simulink model "ML_receiver"  (R2016b)
settings: Solver=VariableStepDiscrete  StartTime=0.0  StopTime=inf  RelTol=1e-3
values from neighbouring files (symbols this model uses):
  avett = exp(1i*2*pi*[0:M-1]/M)    [ML_receiver_matlab.m]
  M = 8    [ML_receiver_matlab.m]    (also in MSE_matlab2.m = 16; OFDM1.m = 64; adaptive_equalization.m = 16)
  T = 1    [ML_receiver_matlab.m]    (also in optimum_filter3.m)
  W = 100/T    (= 100)    [ML_receiver_matlab.m]
libraries: commchan3 x1, commsink2 x1, commrandsrc3 x1, dspstat3 x1, simulink x1
settings Model: Creator=Shu  LastModifiedBy=Shu
settings DataIOCC: LimitDataPoints=on  SaveOutput=off  SaveTime=off
settings OptimizationCC: BooleanDataType=off  DefaultParameterBehavior=Inlined  LocalBlockOutputs=off  LifeSpan=inf
settings DebuggingCC: AlgebraicLoopMsg=error  MultiTaskRateTransMsg=warning  AllowSymbolicDim=off  SFUnexpectedBacktrackingDiag=warning  SFNoUnconditionalDefaultTransitionDiag=warning  SFExecutionAtInitializationDiag=none
settings GRTTargetCC: TargetLangStandard=C89/C90 (ANSI)  GeneratePreprocessorConditionals=Disable all
settings ConfigComp: CovMetricSettings=dw  CovHtmlReporting=on  CovSaveCumulativeToWorkspaceVar=on  CovSaveSingleToWorkspaceVar=on  CovExternalEMLEnable=off  CovSFcnEnable=off

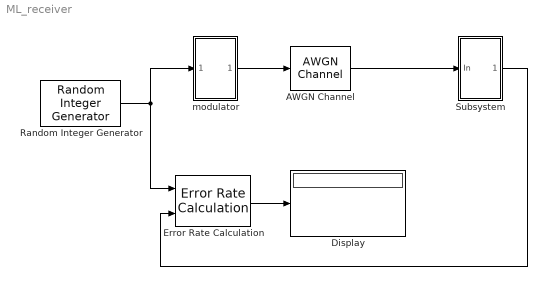
== system ML_receiver ==
  AWGN Channel : commchan3/AWGN Channel  InputProcessing=Columns as channels (frame based)  seed=67  noiseMode="Signal to noise ratio  (Es/No)"  EbNodB=10  EsNodB=SNRdB  SNRdB=SNRdB  bitsPerSym=1  Ps=1  Tsym=1  variance=1
  Display : Display
  Error Rate Calculation : commsink2/Error Rate Calculation  N=1  st_delay=1  cp_mode=Select samples from mask  subframe=[]  PMode=Port  WsName=ErrorVec  RsMode2=off  stop=off  numErr=100  maxBits=1e6
  Random Integer Generator : commrandsrc3/Random Integer Generator  SetSize=M  SeedSource=Auto  Seed=0  SampleTime=T  SamplesPerFrame=1  OutputDataType=double  SimulateUsing=Interpreted execution
  Subsystem : Subsystem
  "modulator " : Subsystem
  wires:
  Random Integer Generator/1 -> Error Rate Calculation/1, "modulator "/1(In1)
  Subsystem/1(Out1) -> Error Rate Calculation/2
  "modulator "/1(Out1) -> AWGN Channel/1
  AWGN Channel/1 -> Subsystem/1(In)
  Error Rate Calculation/1 -> Display/1

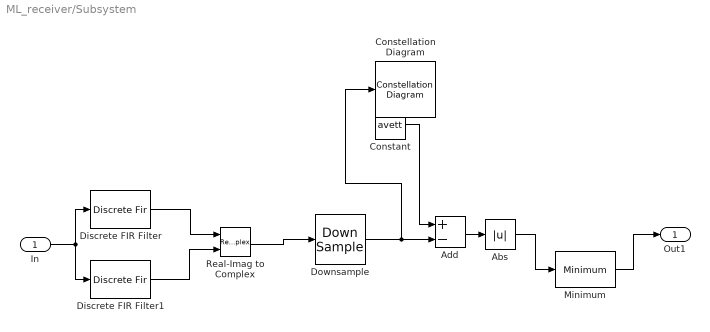
== system ML_receiver/Subsystem ==
  In : Inport
  Abs : Abs
  Add : Sum  Inputs=+-
  Constant : Constant  Value=avett  SampleTime=T
  Constellation Diagram : ConstellationDiagram
  Discrete FIR Filter : DiscreteFir  Coefficients=-sqrt(2/T)*cos(2*pi*((-W+1):0)/W)/W  InputProcessing=Columns as channels (frame based)
  Discrete FIR Filter1 : DiscreteFir  Coefficients=-sqrt(2/T)*sin(2*pi*((-W+1):0)/W)/W  InputProcessing=Columns as channels (frame based)
  Downsample : DownSample  N=W  phase=W-1  RateOptions=Allow multirate processing
  Minimum : dspstat3/Minimum  operation=minimum  fcn=Index  indexBase=Zero  operateOver=Each column  Dimension=1  InputProcessing=Columns as channels (frame based)  reset=None  roiEnable=off  roiType=Rectangles  roiPortion=Entire ROI  roiOutput=Individual statistics for each ROI  roiFlag=off  roundingMode=Floor  overflowMode=off
  Real-Imag to Complex : RealImagToComplex
  Out1 : Outport
  wires:
  In/1 -> Discrete FIR Filter1/1, Discrete FIR Filter/1
  Real-Imag to Complex/1 -> Downsample/1
  Discrete FIR Filter/1 -> Real-Imag to Complex/1
  Discrete FIR Filter1/1 -> Real-Imag to Complex/2
  Downsample/1 -> Constellation Diagram/1, Add/2
  Constant/1 -> Add/1
  Add/1 -> Abs/1
  Abs/1 -> Minimum/1
  Minimum/1 -> Out1/1

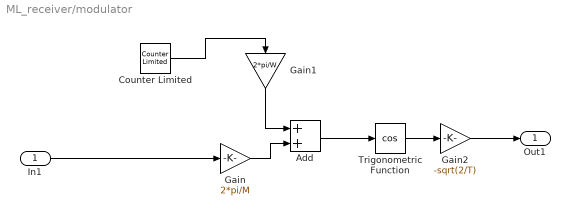
== system ML_receiver/modulator  ==
  In1 : Inport
  Add : Sum
  Counter Limited : simulink/Sources/Counter Limited  uplimit=W-1  tsamp=T/W
  Gain : Gain  Gain=2*pi/M
  Gain1 : Gain  Gain=2*pi/W
  Gain2 : Gain  Gain=-sqrt(2/T)
  Trigonometric Function : Trigonometry  Operator=cos
  Out1 : Outport
  wires:
  In1/1 -> Gain/1
  Trigonometric Function/1 -> Gain2/1
  Gain2/1 -> Out1/1
  Gain1/1 -> Add/1
  Gain/1 -> Add/2
  Add/1 -> Trigonometric Function/1
  Counter Limited/1 -> Gain1/1
